simulink subsystem "Neuron_Subsystem"  (R2025b)
settings: Solver=VariableStepAuto  StartTime=0.0  StopTime=10.0  RelTol=1e-3
settings Model: Creator=chipherzero  LastModifiedBy=chipher

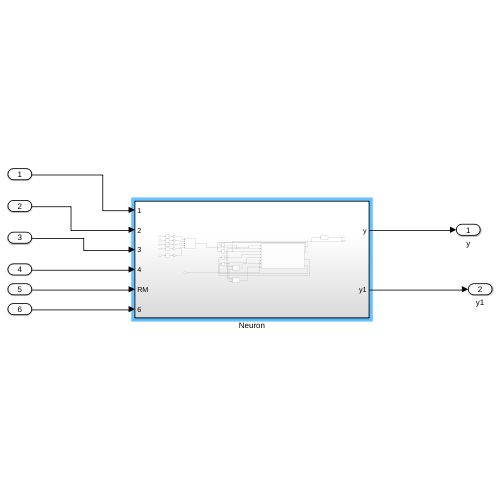
[thumbnail: Simulink's stored preview of the top-level diagram]
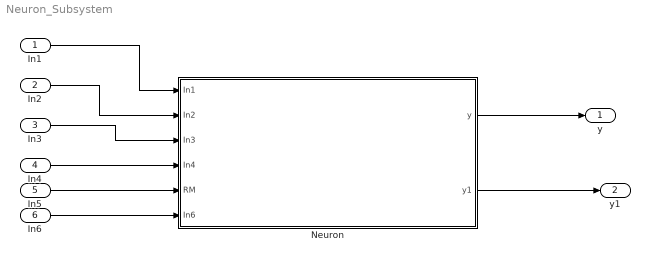
== system Neuron_Subsystem ==
  In1 : Inport
  In2 : Inport  Port=2
  In3 : Inport  Port=3
  In4 : Inport  Port=4
  In5 : Inport  Port=5
  In6 : Inport  Port=6
  Neuron : Subsystem
  y : Outport
  y1 : Outport  Port=2
  wires:
  In1/1 -> Neuron/1(In1)
  In2/1 -> Neuron/2(In2)
  In3/1 -> Neuron/3(In3)
  In4/1 -> Neuron/4(In4)
  In5/1 -> Neuron/5(RM)
  In6/1 -> Neuron/6(In6)
  Neuron/1(y) -> y/1
  Neuron/2(y1) -> y1/1

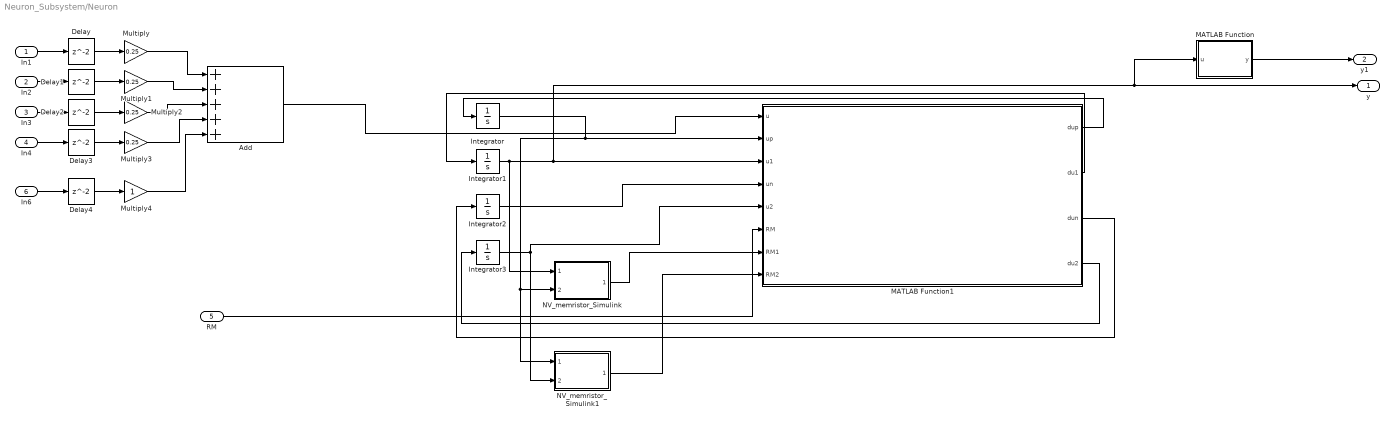
== system Neuron_Subsystem/Neuron ==
  In1 : Inport
  In2 : Inport  Port=2
  In3 : Inport  Port=3
  In4 : Inport  Port=4
  RM : Inport  Port=5
  In6 : Inport  Port=6
  Add : Sum  Inputs=+++++
  Delay{,1..4} (5 alike) : Delay
  Integrator : Integrator
  Integrator1 : Integrator
  Integrator2 : Integrator
  Integrator3 : Integrator  InitialCondition=6e-09
  MATLAB Function : MATLAB Function  TreatAsAtomicUnit=on
  MATLAB Function1 : MATLAB Function  TreatAsAtomicUnit=on
  Multiply{,1..3} (4 alike) : Gain  Gain=0.25
  Multiply4 : Gain
  NV_memristor_Simulink : Subsystem  ReferencedSubsystem=NV_memristor_Simulink
  NV_memristor_Simulink1 : Subsystem  ReferencedSubsystem=NV_memristor_Simulink
  y : Outport
  y1 : Outport  Port=2
  wires:
  Integrator2/1 -> MATLAB Function1/4(un)
  In4/1 -> Delay3/1
  Add/1 -> MATLAB Function1/1(u)
  MATLAB Function1/4(du2) -> Integrator3/1
  NV_memristor_Simulink1/1 -> MATLAB Function1/8(RM2)
  Multiply/1 -> Add/1
  In6/1 -> Delay4/1
  MATLAB Function/1(y) -> y1/1
  Integrator3/1 -> NV_memristor_Simulink1/2, MATLAB Function1/5(u2)
  In3/1 -> Delay2/1
  RM/1 -> MATLAB Function1/6(RM)
  Integrator1/1 -> NV_memristor_Simulink/1, y/1, MATLAB Function/1(u), MATLAB Function1/3(u1)
  MATLAB Function1/2(du1) -> Integrator1/1
  Integrator/1 -> MATLAB Function1/2(up), NV_memristor_Simulink1/1, NV_memristor_Simulink/2
  In1/1 -> Delay/1
  MATLAB Function1/1(dup) -> Integrator/1
  Multiply1/1 -> Add/2
  NV_memristor_Simulink/1 -> MATLAB Function1/7(RM1)
  In2/1 -> Delay1/1
  Multiply4/1 -> Add/5
  MATLAB Function1/3(dun) -> Integrator2/1
  Multiply3/1 -> Add/4
  Multiply2/1 -> Add/3
  Delay/1 -> Multiply/1
  Delay1/1 -> Multiply1/1
  Delay2/1 -> Multiply2/1
  Delay3/1 -> Multiply3/1
  Delay4/1 -> Multiply4/1

== matlab function Neuron_Subsystem/Neuron/MATLAB Function ==
  data: u input; y output
function y = soft_floor(u)
k = 50;        % sharpness
floor = -0.001;
y = floor + (u-floor).*(0.5 + 0.5*tanh(k*(u-floor)));
end

== matlab function Neuron_Subsystem/Neuron/MATLAB Function1 ==
  data: u input; dup output; up input; u1 input; un input; u2 input; RM input; RM1 input; RM2 input; du1 output; dun output; du2 output
function [dup, du1, dun, du2] = neuronDynamics( ...
    u, up, u1, un, u2, ...
    RM, RM1, RM2)
%#codegen
% Simulink-compatible continuous-time state derivatives for the circuit.
% External Integrators: up, u1, un, u2.
% Only memristor resistances (RM,RM1,RM2) are passed in. All other passives
% and op-amp parameters are defined internally below.

% -------------------- INTERNAL PARAMETERS (edit these) --------------------
% Passives
C   = 10e-9;   % [F]
C1  = 10e-9;   % [F]
C2  = 100e-9;   % [F]
C3  = 100e-9;   % [F]
R   = 100e3;    % [ohm]

% Schmitt divider
R2  = 300e3;  % [ohm]
R3  = 300e3;  % [ohm]

% OpAmp1 (left stage)
A1  = 1000;   % gain
R1  = 300e3;    % [ohm] output impedance (your R1)
V1L = -0.6;   % [V] lower rail
V1H =  0.6;   % [V] upper rail

% OpAmp2 (Schmitt stage)
A2     = 1000;  % gain
Rout2  = 100;   % [ohm] output impedance
V2L    = -0.5;  % [V] lower rail
V2H    =  0.5;  % [V] upper rail
% -------------------------------------------------------------------------

% helpers
k=500;
sat = @(x, lo, hi, k) ...
    0.5*(hi + lo) + 0.5*(hi - lo)*tanh( k*(x - 0.5*(hi + lo)) / (0.5*(hi - lo)) );
%sat = @(x, lo, hi,k) min(hi, max(lo, x));


beta = R3 / (R2 + R3);

% internal op-amp source voltages (before output impedances)
ua = sat(A1 * (up - un), V1L, V1H,k);
ub = sat(A2 * (beta*u2 - u1), V2L, V2H,k);

% 1) u_p node
dup = ( (u - up)/RM + (u1 - up)/RM1 + (u2 - up)/RM2 ) / C;

% 2) use C1*d(u1-un)/dt = un/R to eliminate derivative term in u1 KCL
% 3) u1 node KCL:
% C2*du1 + C1*d(u1-un)/dt + (u1-up)/RM1 + (u1-ua)/R1 = 0
% substitute C1*d(u1-un)/dt = un/R:
du1 = -( (un/R) + (u1 - up)/RM1 + (u1 - ua)/R1 ) / C2;

% 4) from C1*(du1 - dun) = un/R  ->  dun = du1 - un/(R*C1)
dun = du1 - un/(R*C1);

% 5) u2 node:
% C3*du2 = (ub-u2)/Rout2 - u2/(R2+R3) - (u2-up)/RM2
du2 = ( (ub - u2)/Rout2 - u2/(R2 + R3) - (u2 - up)/RM2 ) / C3;

end
